simulink model "hoistSim"  (R2015b)
settings: Solver=VariableStepAuto  StartTime=0.0  StopTime=10.0  RelTol=1e-3
settings Model: Creator=OlgeirMac  LastModifiedBy=OlgeirMac

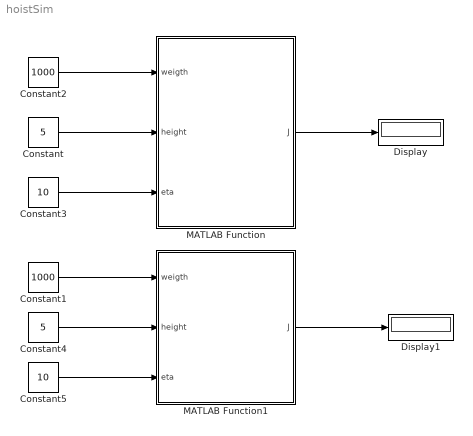
== system hoistSim ==
  Constant : Constant  Value=5
  Constant1 : Constant  Value=1000
  Constant2 : Constant  Value=1000
  Constant3 : Constant  Value=10
  Constant4 : Constant  Value=5
  Constant5 : Constant  Value=10
  Display : Display
      settings: Decimation=3
  Display1 : Display
      settings: Decimation=3
  MATLAB Function : MATLAB Function  TreatAsAtomicUnit=on
  MATLAB Function1 : MATLAB Function  TreatAsAtomicUnit=on
  wires:
  MATLAB Function/1(J) -> Display/1
  MATLAB Function1/1(J) -> Display1/1
  Constant2/1 -> MATLAB Function/1(weigth)
  Constant/1 -> MATLAB Function/2(height)
  Constant3/1 -> MATLAB Function/3(eta)
  Constant1/1 -> MATLAB Function1/1(weigth)
  Constant4/1 -> MATLAB Function1/2(height)
  Constant5/1 -> MATLAB Function1/3(eta)

== matlab function hoistSim/MATLAB Function1 ==
  data: weigth input; J output; height input; eta input
function J  = lowerLoadSim(weigth, height, eta)
    % The function calculates the amount of energy released from the 
    % lowering operation. It takes the weigth that is to be lowered, the
    % heigth it is lowered and eta is the effiency of the system. Effiency in this
    % case means the energy that is released in a controlled manner (in
    % contrary to unspecified friction etc.). The function returns the
    % energy released. SI units i assumed.
    
    Ep = potentialEnergy(weigth,height);    % The potential energy
    
    lower = Ep*eta;     % Calculates how much energy that is released with 
                        % respect taken to the effiency of the system.
    J = lower;
end

== matlab function hoistSim/MATLAB Function ==
  data: weigth input; J output; height input; eta input
function J  = hoistLoadSim(weigth, height, eta)
    % The function calculates the amount of energy used for the hoisting
    % operation. It takes the lifting weigth, the lifting heigth and the
    % efficiency for the whole system as input parameters (including
    % electric motor, friction etc.). The output is energy, and it is with
    % negative sign since the hoisting operation takes energy from one
    % source and store it as potential energy in the container. SI unit is
    % assumed.
    
    Ep = potentialEnergy(weigth,height);    % The potential energy
    
    lift = Ep/eta;     % Calculates how much energy that is needed with 
                       % respect taken to the effiency of the system.
                                          
    J = -lift;
end
